simulink model "AMBD_GlucoMeter_V2"  (R2022a)
settings: Solver=VariableStepAuto  StartTime=0.0  StopTime=10.0  RelTol=1e-3
libraries: simulink x4
settings Model: Creator=yashb  LastModifiedBy=yashb

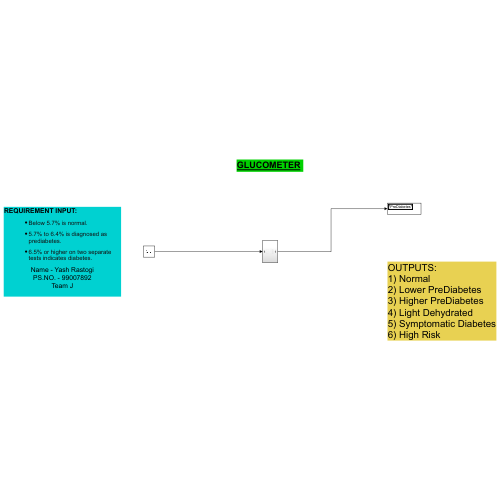
[thumbnail: Simulink's stored preview of the top-level diagram]
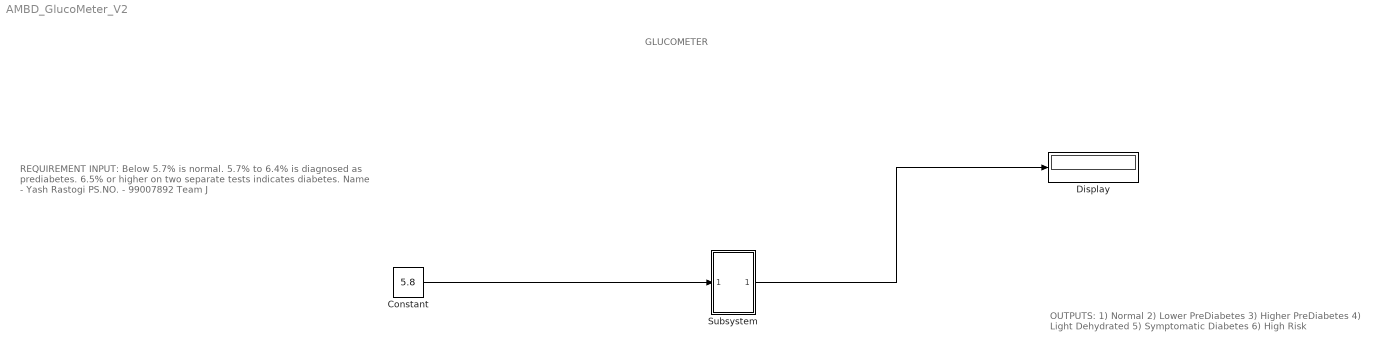
== system AMBD_GlucoMeter_V2 ==
  note: GLUCOMETER
  note: OUTPUTS:
      | 1) Normal
      | 2) Lower PreDiabetes
      | 3) Higher PreDiabetes
      | 4) Light Dehydrated
      | 5) Symptomatic Diabetes
      | 6) High Risk
  note: REQUIREMENT INPUT:
      |
      | Below 5.7% is normal.
      | 5.7% to 6.4% is diagnosed as prediabetes.
      | 6.5% or higher on two separate tests indicates diabetes.
      | Name - Yash Rastogi
      | PS.NO. - 99007892
      | Team J
  Constant : Constant  Value=5.8
  Display : Display
  Subsystem : Subsystem
  wires:
  Constant/1 -> Subsystem/1(In1)
  Subsystem/1(Out1) -> Display/1

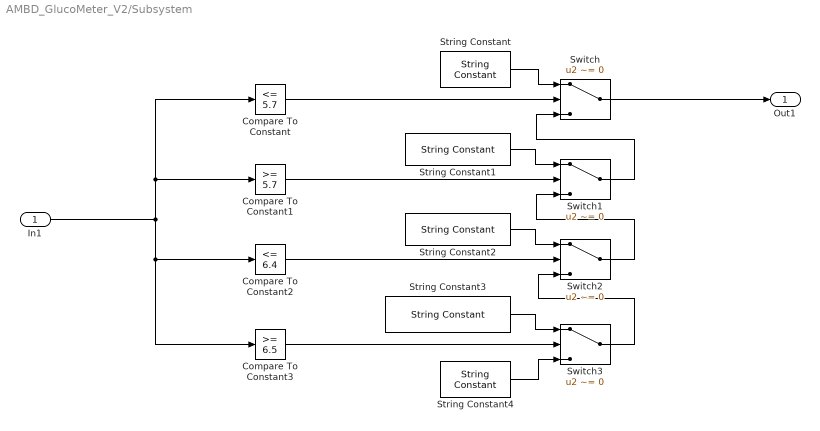
== system AMBD_GlucoMeter_V2/Subsystem ==
  In1 : Inport
  Compare To Constant : simulink/Logic and Bit Operations/Compare To Constant  relop=<=  const=5.7  OutDataTypeStr=boolean
  Compare To Constant1 : simulink/Logic and Bit Operations/Compare To Constant  relop=>=  const=5.7  OutDataTypeStr=boolean
  Compare To Constant2 : simulink/Logic and Bit Operations/Compare To Constant  relop=<=  const=6.4  OutDataTypeStr=boolean
  Compare To Constant3 : simulink/Logic and Bit Operations/Compare To Constant  relop=>=  const=6.5  OutDataTypeStr=boolean
  String Constant : StringConstant  String="\"Normal\""
  String Constant1 : StringConstant  String="\"Lower PreDiabetes\""
  String Constant2 : StringConstant  String="\"Higher PreDiabetes\""
  String Constant3 : StringConstant  String="\"Symptomatic Diabetes\""
  String Constant4 : StringConstant  String="\"High Risk\""
  Switch{,1..3} (4 alike) : Switch  Criteria=u2 ~= 0  SaturateOnIntegerOverflow=off  InputSameDT=off
  Out1 : Outport
  wires:
  In1/1 -> Compare To Constant3/1, Compare To Constant2/1, Compare To Constant1/1, Compare To Constant/1
  Switch2/1 -> Switch1/3
  String Constant4/1 -> Switch3/3
  Compare To Constant3/1 -> Switch3/2
  Switch3/1 -> Switch2/3
  Compare To Constant2/1 -> Switch2/2
  Switch1/1 -> Switch/3
  Compare To Constant/1 -> Switch/2
  Compare To Constant1/1 -> Switch1/2
  String Constant2/1 -> Switch2/1
  Switch/1 -> Out1/1
  String Constant1/1 -> Switch1/1
  String Constant/1 -> Switch/1
  String Constant3/1 -> Switch3/1
